simulink model "real"  (R2014b)
settings: Solver=ode4  StartTime=0.0  StopTime=inf  FixedStep=0.001  RelTol=1e-3
undefined symbols (not defined in the file or in its folder): Advantech, PCI
libraries: rtwinlib x2
settings Model: SimulationMode=external  ExtModeTrigDuration=200000  Creator=Administrator  LastModifiedBy=nk
settings DataIOCC: SignalLoggingSaveFormat=ModelDataLogs
settings OptimizationCC: ExpressionDepthLimit=2147483647  InitFltsAndDblsToZero=on
settings DebuggingCC: SaveWithParameterizedLinksMsg=none  UnderspecifiedInitializationDetection=Classic  MergeDetectMultiDrivingBlocksExec=none  SignalResolutionControl=TryResolveAllWithWarning  MultiTaskDSMMsg=warning  MultiTaskCondExecSysMsg=none  FcnCallInpInsideContextMsg=UseLocalSettings  StateNameClashWarn=warning
settings RTWCC: SystemTargetFile=rtwin.tlc  TemplateMakefile=rtwin.tmf  Description=Real-Time Windows Target  ProcessScript=rtwin_make_rtw_hook  IncludeERTFirstTime=on
settings RTWinTargetCC: TargetFcnLib=ansi_tfl_tmw.mat  TargetLibSuffix=_rtwin.lib  TargetPreCompLibLocation=C:\Program Files\MATLAB\R2014b\toolbox\rtw\targets\rtwin\lib\win64  ModelReferenceCompliant=off  CompOptLevelCompliant=off

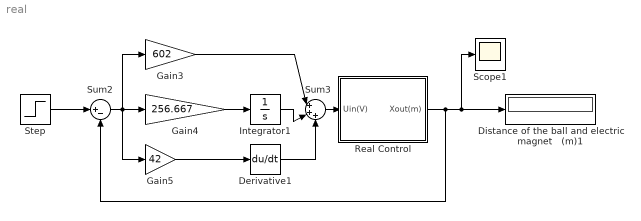
== system real ==
  Derivative1 : Derivative
  Distance of the ball and electric magnet   (m)1 : Display
      settings: Decimation=50
  Gain3 : Gain  Gain=602
  Gain4 : Gain  Gain=256.667
  Gain5 : Gain  Gain=42
  Integrator1 : Integrator
  Real Control : Subsystem
  Scope1 : Scope
  Step : Step  After=-0.01  SampleTime=0
  Sum2 : Sum  Inputs=|+-
  Sum3 : Sum  Inputs=|+++
  wires:
  Real Control/1(Xout(m)) -> Scope1/1, Distance of the ball and electric magnet   (m)1/1, Sum2/2
  Step/1 -> Sum2/1
  Gain4/1 -> Integrator1/1
  Sum2/1 -> Gain4/1, Gain5/1, Gain3/1
  Gain5/1 -> Derivative1/1
  Sum3/1 -> Real Control/1(Uin(V))
  Integrator1/1 -> Sum3/2
  Derivative1/1 -> Sum3/3
  Gain3/1 -> Sum3/1

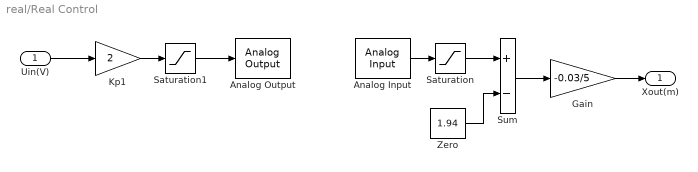
== system real/Real Control ==
  Uin(V) : Inport
  Analog Input : rtwinlib/Analog Input  SampleTime=0.001  MaxMissedTicks=10  ShowMissedTicks=off  YieldWhenWaiting=off  DrvName=Advantech/PCI-1711  DrvAddress=4294967295  DrvOptions=zeros(1,0)  Channels=1  RangeMode=1  VoltRange=2  DataType=1
      settings: AttributesFormatString=Advantech\nPCI-1711 [auto]
  Analog Output : rtwinlib/Analog Output  SampleTime=0.001  MaxMissedTicks=10  ShowMissedTicks=off  YieldWhenWaiting=off  DrvName=Advantech/PCI-1711  DrvAddress=4294967295  DrvOptions=zeros(1,0)  Channels=1  RangeMode=1  VoltRange=2  InitialValue=-10  FinalValue=-10
      settings: AttributesFormatString=Advantech\nPCI-1711 [auto]
  Gain : Gain  Gain=-0.03/5  SaturateOnIntegerOverflow=on  OutDataTypeStr=Inherit: Same as input  ParamDataTypeStr=Inherit: Same as input
  Kp1 : Gain  Gain=2  SaturateOnIntegerOverflow=on  OutDataTypeStr=Inherit: Same as input  ParamDataTypeStr=Inherit: Same as input
  Saturation : Saturate  UpperLimit=5  LowerLimit=0
  Saturation1 : Saturate  UpperLimit=10  LowerLimit=0
  Sum : Sum  Inputs=+-  SaturateOnIntegerOverflow=on  OutDataTypeStr=Inherit: Same as first input
  Zero : Constant  Value=1.94  SampleTime=-1
  Xout(m) : Outport
  wires:
  Gain/1 -> Xout(m)/1
  Zero/1 -> Sum/2
  Sum/1 -> Gain/1
  Saturation/1 -> Sum/1
  Analog Input/1 -> Saturation/1
  Kp1/1 -> Saturation1/1
  Uin(V)/1 -> Kp1/1
  Saturation1/1 -> Analog Output/1
